simulink model "default_model"  (R2023b)
settings: Solver=VariableStepAuto  StartTime=0.0  StopTime=2000  RelTol=1e-3
model workspace (MAT data in the model file):
  Cd = 180
  Csh = 30
  K = 3.1616
  Tauf = 5
  Tf = 8
  Tfuel = 8
  Tw = 6
  k = 3.1616
settings Model: Creator=jakub  LastModifiedBy=jakub

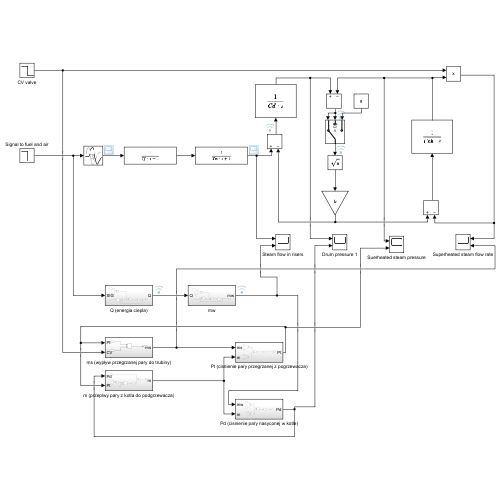
[thumbnail: Simulink's stored preview of the top-level diagram]
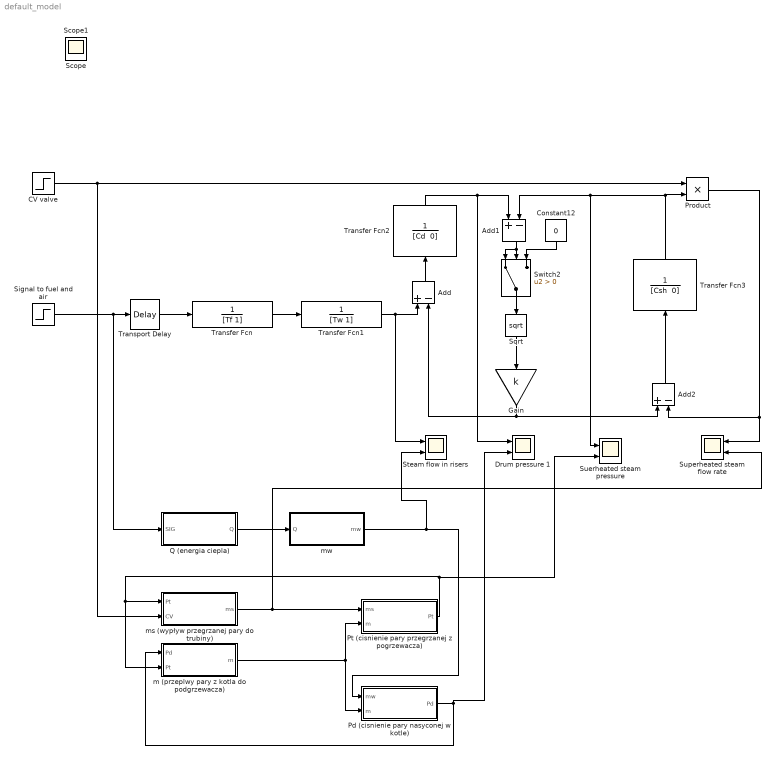
== system default_model ==
  " mw " : Subsystem
  Add : Sum  Inputs=+-
  Add1 : Sum  Inputs=+-
  Add2 : Sum  Inputs=+-
  CV valve : Step  Before=1  After=0  SampleTime=0
  Constant12 : Constant  Value=0
  Drum pressure 1 : Scope  NumInputPorts=2
  Gain : Gain  Gain=k
  Pd (cisnienie pary nasyconej w kotle) : Subsystem
  Product : Product
  Pt (cisnienie pary przegrzanej z pogrzewacza) : Subsystem
  Q (energia ciepla) : Subsystem
  Signal to fuel and air : Step  Before=1  After=0  SampleTime=0
  Sqrt : Sqrt
  Steam flow in risers : Scope  NumInputPorts=2
  Suerheated steam pressure : Scope  NumInputPorts=2
  Superheated steam flow rate : Scope  NumInputPorts=2
  Switch2 : Switch  Criteria=u2 > Threshold  SaturateOnIntegerOverflow=off  InputSameDT=off
  Transfer Fcn : TransferFcn  Denominator=[Tf 1]
  Transfer Fcn1 : TransferFcn  Denominator=[Tw 1]
  Transfer Fcn2 : TransferFcn  Denominator="[Cd  0]"
  Transfer Fcn3 : TransferFcn  Denominator="[Csh  0]"
  Transport Delay : TransportDelay  DelayTime=Tauf
  m (przeplwy pary z kotla do podgrzewacza) : Subsystem
  ms (wypływ przegrzanej pary do trubiny) : Subsystem
  Scope : Scope
  Scope1 : Scope
  wires:
  Transfer Fcn3/1 -> Suerheated steam pressure/1, Add1/2, Product/2
  Add2/1 -> Transfer Fcn3/1
  Product/1 -> Superheated steam flow rate/1, Add2/2
  Gain/1 -> Add2/1, Add/2
  CV valve/1 -> Product/1, ms (wypływ przegrzanej pary do trubiny)/2(CV)
  Transport Delay/1 -> Transfer Fcn/1
  Signal to fuel and air/1 -> Q (energia ciepla)/1(SIG), Transport Delay/1
  Transfer Fcn2/1 -> Drum pressure 1/1, Add1/1
  Transfer Fcn1/1 -> Steam flow in risers/1, Add/1
  Add/1 -> Transfer Fcn2/1
  Sqrt/1 -> Gain/1
  Transfer Fcn/1 -> Transfer Fcn1/1
  Q (energia ciepla)/1(Q) -> " mw "/1(Q)
  ms (wypływ przegrzanej pary do trubiny)/1(ms) -> Superheated steam flow rate/2, Pt (cisnienie pary przegrzanej z pogrzewacza)/1(ms)
  Pt (cisnienie pary przegrzanej z pogrzewacza)/1(Pt) -> Suerheated steam pressure/2, ms (wypływ przegrzanej pary do trubiny)/1(Pt), m (przeplwy pary z kotla do podgrzewacza)/2(Pt)
  m (przeplwy pary z kotla do podgrzewacza)/1(m) -> Pd (cisnienie pary nasyconej w kotle)/2(m), Pt (cisnienie pary przegrzanej z pogrzewacza)/2(m)
  " mw "/1(mw) -> Steam flow in risers/2, Pd (cisnienie pary nasyconej w kotle)/1(mw)
  Pd (cisnienie pary nasyconej w kotle)/1(Pd) -> m (przeplwy pary z kotla do podgrzewacza)/1(Pd), Drum pressure 1/2
  Add1/1 -> Switch2/1, Switch2/2
  Switch2/1 -> Sqrt/1
  Constant12/1 -> Switch2/3

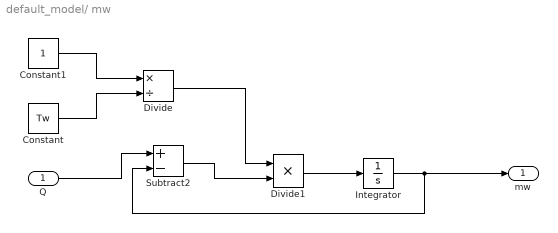
== system default_model/ mw  ==
  Q : Inport
  Constant : Constant  Value=Tw
  Constant1 : Constant
  Divide : Product  Inputs=*/
  Divide1 : Product  Inputs=**  RndMeth=Zero  SaturateOnIntegerOverflow=on
  Integrator : Integrator
  Subtract2 : Sum  Inputs=+-
  mw : Outport
  wires:
  Divide/1 -> Divide1/1
  Constant1/1 -> Divide/1
  Constant/1 -> Divide/2
  Divide1/1 -> Integrator/1
  Integrator/1 -> Subtract2/2, mw/1
  Q/1 -> Subtract2/1
  Subtract2/1 -> Divide1/2

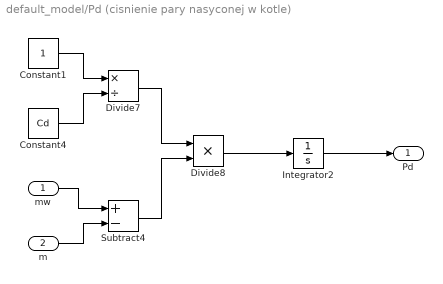
== system default_model/Pd (cisnienie pary nasyconej w kotle) ==
  mw : Inport
  m : Inport  Port=2
  Constant1 : Constant
  Constant4 : Constant  Value=Cd
  Divide7 : Product  Inputs=*/
  Divide8 : Product  Inputs=**
  Integrator2 : Integrator
  Subtract4 : Sum  Inputs=+-
  Pd : Outport
  wires:
  mw/1 -> Subtract4/1
  m/1 -> Subtract4/2
  Constant4/1 -> Divide7/2
  Constant1/1 -> Divide7/1
  Subtract4/1 -> Divide8/2
  Divide7/1 -> Divide8/1
  Divide8/1 -> Integrator2/1
  Integrator2/1 -> Pd/1

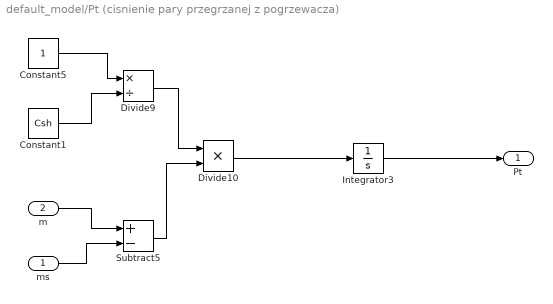
== system default_model/Pt (cisnienie pary przegrzanej z pogrzewacza) ==
  ms : Inport
  m : Inport  Port=2
  Constant1 : Constant  Value=Csh
  Constant5 : Constant
  Divide10 : Product  Inputs=**
  Divide9 : Product  Inputs=*/
  Integrator3 : Integrator
  Subtract5 : Sum  Inputs=+-
  Pt : Outport
  wires:
  ms/1 -> Subtract5/2
  m/1 -> Subtract5/1
  Constant1/1 -> Divide9/2
  Constant5/1 -> Divide9/1
  Divide9/1 -> Divide10/1
  Subtract5/1 -> Divide10/2
  Divide10/1 -> Integrator3/1
  Integrator3/1 -> Pt/1

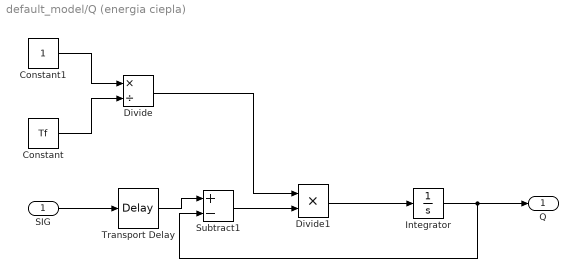
== system default_model/Q (energia ciepla) ==
  SIG : Inport
  Constant : Constant  Value=Tf
  Constant1 : Constant
  Divide : Product  Inputs=*/
  Divide1 : Product  Inputs=**  RndMeth=Zero  SaturateOnIntegerOverflow=on
  Integrator : Integrator
  Subtract1 : Sum  Inputs=+-
  Transport Delay : TransportDelay  DelayTime=Tauf
  Q : Outport
  wires:
  SIG/1 -> Transport Delay/1
  Transport Delay/1 -> Subtract1/1
  Subtract1/1 -> Divide1/2
  Constant1/1 -> Divide/1
  Constant/1 -> Divide/2
  Divide/1 -> Divide1/1
  Divide1/1 -> Integrator/1
  Integrator/1 -> Subtract1/2, Q/1

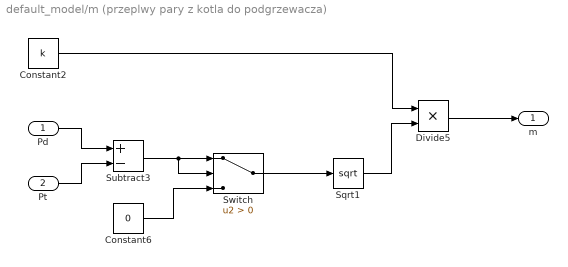
== system default_model/m (przeplwy pary z kotla do podgrzewacza) ==
  Pd : Inport
  Pt : Inport  Port=2
  Constant2 : Constant  Value=k
  Constant6 : Constant  Value=0
  Divide5 : Product  Inputs=**
  Sqrt1 : Sqrt
  Subtract3 : Sum  Inputs=+-
  Switch : Switch  Criteria=u2 > Threshold  SaturateOnIntegerOverflow=off  InputSameDT=off
  m : Outport
  wires:
  Pd/1 -> Subtract3/1
  Pt/1 -> Subtract3/2
  Constant6/1 -> Switch/3
  Subtract3/1 -> Switch/1, Switch/2
  Switch/1 -> Sqrt1/1
  Constant2/1 -> Divide5/1
  Sqrt1/1 -> Divide5/2
  Divide5/1 -> m/1

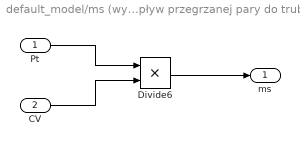
== system default_model/ms (wypływ przegrzanej pary do trubiny) ==
  Pt : Inport
  CV : Inport  Port=2
  Divide6 : Product  Inputs=**
  ms : Outport
  wires:
  Pt/1 -> Divide6/1
  CV/1 -> Divide6/2
  Divide6/1 -> ms/1
